simulink model "Electrical_System_2018b_obfs"  (R2019b)
settings: Solver=VariableStepAuto  StartTime=0.0  StopTime=5  RelTol=1e-3  AbsTol=1e-3  EnableMultiTasking=on
InitFcn:
  | Steady_State_Initialisation;
StopFcn:
  | %sscexplore(simlog);
  | %Logging
undefined symbols (not defined in the file): abrlhklxvp, aexgmhuedq, afmfmjnutg, afpphrjpnc, ahuxbyvruc, alarvljztt, amxnyqmnuw, aodrlwvqie, aolhmuplyq, aqpmguuqkg, auesgwirzl, aurophlnng, awamelrhru, ayfhvxflxn, azxkacuhqc, babszerikg, bawhdqanwq, bevoqecvei, bltjvqbchx, bmqsuewujl, bsmyqjfgnf, btvjbsmnve, bywgxqeadw, bziaduxaer, bzmcmdqocb, bzsvyvetat, ccsjnrbsih, cdvenygxwh, cedkrnslhx, cjheorclzs, cjrdshrtqx, ckhavyhcza, ckxewznhlz, cmrcgyiplk, conenicnws, cqkejbgjnn, csfnuwymhe, cunupkhwbh, cwzfvzuxxh, dcadmadufn, dcfponivnv, ddtrqjrhjn, dfhoxvkqas, dfrhtcwpne, dfvomcagjv, djijwylxea, dnmeqksrrm, dnzewbdkaa, dsqcykyxav, dtswwlttmm, ecumpidjtv, edegaywrct, ejjjsmnejc, eknqnehjdz, emvdetzouf, esxbqkbahr, etnkkbreiq, eunoiiiirw, ewewcuedir, fatkfxdhtc ... (+386)
libraries: fl_lib x802, ee_lib x362, fl_ps_legacy_lib x160, nesl_utility x85
(part 2 of 26)

== system Electrical_System_2018b_obfs/Redacted_1221/Redacted_346/Redacted_6610 ==
  Redacted_3546 : Inport
  Redacted_2515 : SimscapeBus  HierarchyStrings=Redacted_600;Redacted_800;Redacted_9392;Redacted_4467
  Redacted_2835 : Subsystem  VariantControlMode=Label  Variant=on  VariantControl=Variant1  LabelModeActiveChoice=Choice
  Redacted_4977 : SimscapeBus  HierarchyStrings=Redacted_3183
  Redacted_8751 : SimscapeBus  HierarchyStrings=Redacted_4818
  Redacted_9208 : SimscapeBus  HierarchyStrings=Redacted_5646;Redacted_1726
  Redacted_995 : SimscapeBus  HierarchyStrings=Redacted_3018;Redacted_5170;Redacted_146
  Redacted_2253 : PMIOPort  Side=Left
  Redacted_1746 : Outport
  wires:
  Redacted_3546/1 -> Redacted_2835/1(Redacted_1740)
  Redacted_2835/1(Redacted_5993) -> Redacted_1746/1
  connections:
  Redacted_2515/LConn3 -- Redacted_9208/RConn1
  Redacted_2515/LConn1 -- Redacted_4977/RConn1
  Redacted_995/RConn1 -- Redacted_2515/LConn4
  Redacted_2253/RConn1 -- Redacted_2515/RConn1
  Redacted_9208/LConn2 -- Redacted_2835/LConn4
  Redacted_8751/LConn1 -- Redacted_2835/LConn2
  Redacted_2515/LConn2 -- Redacted_8751/RConn1
  Redacted_995/LConn1 -- Redacted_2835/RConn1
  Redacted_9208/LConn1 -- Redacted_2835/LConn3
  Redacted_4977/LConn1 -- Redacted_2835/LConn1
  Redacted_995/LConn3 -- Redacted_2835/RConn3
  Redacted_995/LConn2 -- Redacted_2835/RConn2

== system Electrical_System_2018b_obfs/Redacted_1221/Redacted_7523/Redacted_2432 ==
  Redacted_3217 : Inport
  Redacted_3397 : Subsystem  VariantControlMode=Label  Variant=on  VariantControl=Variant1  LabelModeActiveChoice=Choice
  Redacted_4698 : SimscapeBus  HierarchyStrings=Redacted_3957;Redacted_2283
  Redacted_558 : SimscapeBus  HierarchyStrings=Redacted_3;Redacted_3627
  Redacted_672 : SimscapeBus  HierarchyStrings=Redacted_5659;Redacted_4345;Redacted_6835
  Redacted_3110 : PMIOPort  Side=Left
  Redacted_9205 : Outport
  wires:
  Redacted_3217/1 -> Redacted_3397/1(Redacted_7824)
  Redacted_3397/1(Redacted_3107) -> Redacted_9205/1
  connections:
  Redacted_672/LConn1 -- Redacted_3397/RConn1
  Redacted_3397/LConn2 -- Redacted_558/LConn2
  Redacted_672/LConn3 -- Redacted_3397/RConn3
  Redacted_3397/LConn1 -- Redacted_558/LConn1
  Redacted_672/LConn2 -- Redacted_3397/RConn2
  Redacted_4698/LConn1 -- Redacted_558/RConn1
  Redacted_4698/LConn2 -- Redacted_672/RConn1
  Redacted_4698/RConn1 -- Redacted_3110/RConn1

== system Electrical_System_2018b_obfs/Redacted_1221/Redacted_7523/Redacted_5456 ==
  Redacted_8021 : Inport
  Redacted_1170 : Subsystem  VariantControlMode=Label  Variant=on  VariantControl=Variant1  LabelModeActiveChoice=Choice
  Redacted_1204 : SimscapeBus  HierarchyStrings=Redacted_6397
  Redacted_2158 : SimscapeBus  HierarchyStrings=Redacted_1826;Redacted_8420;Redacted_7159
  Redacted_6920 : SimscapeBus  HierarchyStrings=Redacted_4449;Redacted_3882
  Redacted_8170 : SimscapeBus  HierarchyStrings=Redacted_9228
  Redacted_9627 : SimscapeBus  HierarchyStrings=Redacted_8942;Redacted_3488;Redacted_7360;Redacted_9767
  Redacted_2988 : PMIOPort  Side=Left
  Redacted_3690 : Outport
  wires:
  Redacted_8021/1 -> Redacted_1170/1(Redacted_533)
  Redacted_1170/1(Redacted_7763) -> Redacted_3690/1
  connections:
  Redacted_9627/RConn1 -- Redacted_2988/RConn1
  Redacted_1170/LConn3 -- Redacted_6920/LConn1
  Redacted_1170/RConn2 -- Redacted_2158/LConn2
  Redacted_1170/LConn1 -- Redacted_8170/LConn1
  Redacted_1170/RConn3 -- Redacted_2158/LConn3
  Redacted_1170/LConn2 -- Redacted_1204/LConn1
  Redacted_1170/RConn1 -- Redacted_2158/LConn1
  Redacted_1170/LConn4 -- Redacted_6920/LConn2
  Redacted_9627/LConn1 -- Redacted_8170/RConn1
  Redacted_9627/LConn2 -- Redacted_1204/RConn1
  Redacted_9627/LConn3 -- Redacted_6920/RConn1
  Redacted_2158/RConn1 -- Redacted_9627/LConn4

== system Electrical_System_2018b_obfs/Redacted_1221/Redacted_7523/Redacted_5495 ==
  Redacted_4129 : Inport
  Redacted_1590 : SimscapeBus  HierarchyStrings=Redacted_4201;Redacted_9003;Redacted_1739;Redacted_5428
  Redacted_2272 : SimscapeBus  HierarchyStrings=Redacted_9234
  Redacted_2383 : SimscapeBus  HierarchyStrings=Redacted_6746;Redacted_4242;Redacted_8
  Redacted_794 : Subsystem  VariantControlMode=Label  Variant=on  VariantControl=Variant1  LabelModeActiveChoice=Choice
  Redacted_8177 : SimscapeBus  HierarchyStrings=Redacted_1099
  Redacted_9332 : SimscapeBus  HierarchyStrings=Redacted_5631;Redacted_7132
  Redacted_391 : PMIOPort  Side=Left
  Redacted_3176 : Outport
  wires:
  Redacted_4129/1 -> Redacted_794/1(Redacted_2518)
  Redacted_794/1(Redacted_6500) -> Redacted_3176/1
  connections:
  Redacted_1590/LConn3 -- Redacted_9332/RConn1
  Redacted_1590/LConn1 -- Redacted_2272/RConn1
  Redacted_2383/RConn1 -- Redacted_1590/LConn4
  Redacted_391/RConn1 -- Redacted_1590/RConn1
  Redacted_9332/LConn2 -- Redacted_794/LConn4
  Redacted_8177/LConn1 -- Redacted_794/LConn2
  Redacted_1590/LConn2 -- Redacted_8177/RConn1
  Redacted_2383/LConn1 -- Redacted_794/RConn1
  Redacted_9332/LConn1 -- Redacted_794/LConn3
  Redacted_2272/LConn1 -- Redacted_794/LConn1
  Redacted_2383/LConn3 -- Redacted_794/RConn3
  Redacted_2383/LConn2 -- Redacted_794/RConn2

== system Electrical_System_2018b_obfs/Redacted_1221/Redacted_7523/Redacted_6578 ==
  Redacted_753 : Inport
  Redacted_3467 : SimscapeBus  HierarchyStrings=Redacted_171;Redacted_7854
  Redacted_4285 : Subsystem  VariantControlMode=Label  Variant=on  VariantControl=Variant1  LabelModeActiveChoice=Variant1
  Redacted_6843 : SimscapeBus  HierarchyStrings=Redacted_6362;Redacted_5590;Redacted_3762;Redacted_3483;Redacted_686;Redacted_7306;Redacted_1915;Redacted_3972
  Redacted_8097 : SimscapeBus  HierarchyStrings=Redacted_6918;Redacted_8095
  Redacted_3223 : PMIOPort  Side=Left
  Redacted_9705 : Outport
  wires:
  Redacted_753/1 -> Redacted_4285/1(Redacted_4594)
  Redacted_4285/1(Redacted_2646) -> Redacted_9705/1
  connections:
  Redacted_4285/LConn5 -- Redacted_6843/LConn6
  Redacted_3467/LConn1 -- Redacted_4285/LConn1
  Redacted_4285/LConn3 -- Redacted_6843/LConn8
  Redacted_6843/LConn2 -- Redacted_4285/RConn2
  Redacted_4285/LConn6 -- Redacted_6843/LConn5
  Redacted_3467/LConn2 -- Redacted_4285/LConn2
  Redacted_4285/LConn4 -- Redacted_6843/LConn7
  Redacted_6843/LConn1 -- Redacted_4285/RConn1
  Redacted_6843/LConn3 -- Redacted_4285/RConn3
  Redacted_4285/RConn4 -- Redacted_6843/LConn4
  Redacted_8097/LConn2 -- Redacted_6843/RConn1
  Redacted_8097/LConn1 -- Redacted_3467/RConn1
  Redacted_8097/RConn1 -- Redacted_3223/RConn1

== system Electrical_System_2018b_obfs/Redacted_1221/Redacted_7996/Redacted_1 ==
  Redacted_5759 : Inport
  Redacted_2550 : SimscapeBus  HierarchyStrings=Redacted_9618;Redacted_4736
  Redacted_3408 : SimscapeBus  HierarchyStrings=Redacted_1645;Redacted_1267;Redacted_9239;Redacted_9750;Redacted_2245;Redacted_273;Redacted_7118;Redacted_512;Redacted_9809;Redacted_8655;Redacted_936;Redacted_8903;Redacted_7027;Redacted_2453;Redacted_972;Redacted_5288;Redacted_8936;Redacted_9531;Redacted_1783;Redacted_8874;Redacted_9030;Redacted_9120;Redacted_4250;Redacted_7101;Redacted_1578;Redacted_9542;Redacted_8423;Redacted_564;Redacted_4281;Redacted_5468;Redacted_3178;Redacted_328;Redacted_8353;Redacted_293;Redacted_8011;Redacted_7574;Redacted_3943;Redacted_8035;Redacted_1472;Redacted_2571;Redacted_9409;Redacted_7767;Redacted_2428;Redacted_1775;Redacted_6878;Redacted_6039;Redacted_5631;Redacted_9047;Redacted_6076
  Redacted_4377 : Subsystem  VariantControlMode=Label  Variant=on  VariantControl=Variant1  LabelModeActiveChoice=Variant4
  Redacted_8912 : BusSelector  OutputSignals=signal1,signal2,signal3,signal4,signal5,signal6,signal7,signal8,signal9,signal10,signal11,signal12,signal13,signal14,signal15,signal16,signal17,signal18,signal19,signal20,signal21,signal22,signal23,signal24
  Redacted_9300 : SimscapeBus  HierarchyStrings=Redacted_6695;Redacted_8811;Redacted_4024;Redacted_6812;Redacted_1080;Redacted_4478;Redacted_4882;Redacted_900;Redacted_1829;Redacted_7949;Redacted_6769;Redacted_9961;Redacted_3619;Redacted_8591;Redacted_4002;Redacted_4612;Redacted_7888;Redacted_7199;Redacted_4226;Redacted_1876;Redacted_4026;Redacted_5676;Redacted_550;Redacted_3264
  Redacted_9946 : PMIOPort  Side=Left
  Redacted_8821 : PMIOPort  Port=2  Side=Right
  Redacted_8480 : PMIOPort  Port=3  Side=Right
  Redacted_2579 : PMIOPort  Port=4  Side=Right
  Redacted_4777 : Outport
  wires:
  Redacted_8912/13 -> Redacted_4377/13(Redacted_310)  "<signal13>"
  Redacted_8912/14 -> Redacted_4377/14(Redacted_3079)  "<signal14>"
  Redacted_8912/5 -> Redacted_4377/5(Redacted_6798)  "<signal5>"
  Redacted_8912/12 -> Redacted_4377/12(Redacted_6586)  "<signal12>"
  Redacted_8912/6 -> Redacted_4377/6(Redacted_2583)  "<signal6>"
  Redacted_8912/10 -> Redacted_4377/10(Redacted_8855)  "<signal10>"
  Redacted_8912/9 -> Redacted_4377/9(Redacted_970)  "<signal9>"
  Redacted_8912/2 -> Redacted_4377/2(Redacted_5838)  "<signal2>"
  Redacted_8912/16 -> Redacted_4377/16(Redacted_2310)  "<signal16>"
  Redacted_8912/11 -> Redacted_4377/11(Redacted_968)  "<signal11>"
  Redacted_8912/4 -> Redacted_4377/4(Redacted_5102)  "<signal4>"
  Redacted_8912/7 -> Redacted_4377/7(Redacted_1780)  "<signal7>"
  Redacted_5759/1 -> Redacted_8912/1
  Redacted_8912/8 -> Redacted_4377/8(Redacted_5045)  "<signal8>"
  Redacted_8912/3 -> Redacted_4377/3(Redacted_3185)  "<signal3>"
  Redacted_8912/1 -> Redacted_4377/1(Redacted_6515)  "<signal1>"
  Redacted_8912/15 -> Redacted_4377/15(Redacted_2830)  "<signal15>"
  Redacted_8912/17 -> Redacted_4377/17(Redacted_4631)  "<signal17>"
  Redacted_8912/18 -> Redacted_4377/18(Redacted_9555)  "<signal18>"
  Redacted_8912/19 -> Redacted_4377/19(Redacted_7717)  "<signal19>"
  Redacted_8912/20 -> Redacted_4377/20(Redacted_8172)  "<signal20>"
  Redacted_8912/21 -> Redacted_4377/21(Redacted_9013)  "<signal21>"
  Redacted_8912/22 -> Redacted_4377/22(Redacted_7477)  "<signal22>"
  Redacted_8912/23 -> Redacted_4377/23(Redacted_1693)  "<signal23>"
  Redacted_8912/24 -> Redacted_4377/24(Redacted_9125)  "<signal24>"
  connections:
  Redacted_4377/RConn12 -- Redacted_3408/LConn12
  Redacted_4377/RConn7 -- Redacted_3408/LConn7
  Redacted_4377/RConn19 -- Redacted_3408/LConn19
  Redacted_4377/RConn11 -- Redacted_3408/LConn11
  Redacted_4377/RConn28 -- Redacted_3408/LConn28
  Redacted_4377/RConn26 -- Redacted_3408/LConn26
  Redacted_8821/RConn1 -- Redacted_4377/RConn50
  Redacted_4377/RConn27 -- Redacted_3408/LConn27
  Redacted_4377/RConn22 -- Redacted_3408/LConn22
  Redacted_3408/LConn31 -- Redacted_4377/RConn31
  Redacted_4377/RConn29 -- Redacted_3408/LConn29
  Redacted_4377/RConn8 -- Redacted_3408/LConn8
  Redacted_4377/RConn9 -- Redacted_3408/LConn9
  Redacted_4377/RConn6 -- Redacted_3408/LConn6
  Redacted_4377/RConn13 -- Redacted_3408/LConn13
  Redacted_4377/RConn14 -- Redacted_3408/LConn14
  Redacted_4377/RConn24 -- Redacted_3408/LConn24
  Redacted_4377/RConn15 -- Redacted_3408/LConn15
  Redacted_4377/RConn20 -- Redacted_3408/LConn20
  Redacted_4377/RConn10 -- Redacted_3408/LConn10
  Redacted_4377/RConn17 -- Redacted_3408/LConn17
  Redacted_4377/RConn18 -- Redacted_3408/LConn18
  Redacted_4377/RConn16 -- Redacted_3408/LConn16
  Redacted_4377/RConn5 -- Redacted_3408/LConn5
  Redacted_4377/RConn21 -- Redacted_3408/LConn21
  Redacted_3408/LConn30 -- Redacted_4377/RConn30
  Redacted_4377/RConn25 -- Redacted_3408/LConn25
  Redacted_4377/RConn23 -- Redacted_3408/LConn23
  Redacted_4377/RConn52 -- Redacted_2579/RConn1
  Redacted_4377/RConn51 -- Redacted_8480/RConn1
  Redacted_3408/LConn4 -- Redacted_4377/RConn4
  Redacted_3408/LConn2 -- Redacted_4377/RConn2
  Redacted_3408/LConn3 -- Redacted_4377/RConn3
  Redacted_3408/LConn1 -- Redacted_4377/RConn1
  Redacted_3408/RConn1 -- Redacted_2550/LConn2
  Redacted_9946/RConn1 -- Redacted_2550/RConn1
  Redacted_9300/LConn1 -- Redacted_4377/LConn1
  Redacted_9300/LConn2 -- Redacted_4377/LConn2
  Redacted_9300/LConn3 -- Redacted_4377/LConn3
  Redacted_9300/LConn4 -- Redacted_4377/LConn4
  Redacted_9300/LConn5 -- Redacted_4377/LConn5
  Redacted_9300/LConn6 -- Redacted_4377/LConn6
  Redacted_9300/LConn7 -- Redacted_4377/LConn7
  Redacted_9300/LConn8 -- Redacted_4377/LConn8
  Redacted_9300/LConn9 -- Redacted_4377/LConn9
  Redacted_9300/LConn10 -- Redacted_4377/LConn10
  Redacted_9300/LConn11 -- Redacted_4377/LConn11
  Redacted_9300/LConn12 -- Redacted_4377/LConn12
  Redacted_9300/LConn13 -- Redacted_4377/LConn13
  Redacted_9300/LConn14 -- Redacted_4377/LConn14
  Redacted_9300/LConn15 -- Redacted_4377/LConn15
  Redacted_9300/LConn16 -- Redacted_4377/LConn16
  Redacted_2550/LConn1 -- Redacted_9300/RConn1
  Redacted_9300/LConn18 -- Redacted_4377/LConn18
  Redacted_9300/LConn19 -- Redacted_4377/LConn19
  Redacted_9300/LConn17 -- Redacted_4377/LConn17
  Redacted_9300/LConn20 -- Redacted_4377/LConn20
  Redacted_9300/LConn21 -- Redacted_4377/LConn21
  Redacted_9300/LConn22 -- Redacted_4377/LConn22
  Redacted_9300/LConn23 -- Redacted_4377/LConn23
  Redacted_9300/LConn24 -- Redacted_4377/LConn24
  Redacted_3408/LConn32 -- Redacted_4377/RConn32
  Redacted_3408/LConn33 -- Redacted_4377/RConn33
  Redacted_3408/LConn34 -- Redacted_4377/RConn34
  Redacted_3408/LConn35 -- Redacted_4377/RConn35
  Redacted_3408/LConn36 -- Redacted_4377/RConn36
  Redacted_3408/LConn37 -- Redacted_4377/RConn37
  Redacted_3408/LConn38 -- Redacted_4377/RConn38
  Redacted_3408/LConn39 -- Redacted_4377/RConn39
  Redacted_3408/LConn40 -- Redacted_4377/RConn40
  Redacted_3408/LConn41 -- Redacted_4377/RConn41
  Redacted_3408/LConn42 -- Redacted_4377/RConn42
  Redacted_3408/LConn43 -- Redacted_4377/RConn43
  Redacted_3408/LConn44 -- Redacted_4377/RConn44
  Redacted_3408/LConn45 -- Redacted_4377/RConn45
  Redacted_3408/LConn46 -- Redacted_4377/RConn46
  Redacted_3408/LConn47 -- Redacted_4377/RConn47
  Redacted_3408/LConn48 -- Redacted_4377/RConn48
  Redacted_4377/RConn49 -- Redacted_3408/LConn49

== system Electrical_System_2018b_obfs/Redacted_1221/Redacted_7996/Redacted_2 ==
  Redacted_9139 : Inport
  Redacted_2321 : SimscapeBus  HierarchyStrings=Redacted_9740;Redacted_2584
  Redacted_3302 : SimscapeBus  HierarchyStrings=Redacted_3734;Redacted_3790;Redacted_712;Redacted_9760;Redacted_78;Redacted_8266
  Redacted_38 : Subsystem  VariantControlMode=Label  Variant=on  VariantControl=Variant1  LabelModeActiveChoice=Variant1
  Redacted_6014 : SimscapeBus  HierarchyStrings=Redacted_7779;Redacted_9774;Redacted_1058;Redacted_9808;Redacted_661;Redacted_3856;Redacted_607;Redacted_1221;Redacted_8690;Redacted_6084
  Redacted_6226 : BusSelector  OutputSignals=signal25,signal26,signal27,signal28,signal29,signal30
  Redacted_7352 : PMIOPort  Side=Left
  Redacted_3930 : PMIOPort  Port=2  Side=Right
  Redacted_7448 : PMIOPort  Port=3  Side=Right
  Redacted_3058 : PMIOPort  Port=4  Side=Right
  Redacted_9760 : PMIOPort  Port=5  Side=Right
  Redacted_7172 : PMIOPort  Port=6  Side=Right
  Redacted_5489 : PMIOPort  Port=7  Side=Right
  Redacted_9750 : Outport
  wires:
  Redacted_6226/5 -> Redacted_38/5(Redacted_9135)  "<signal29>"
  Redacted_6226/2 -> Redacted_38/2(Redacted_9730)  "<signal26>"
  Redacted_9139/1 -> Redacted_6226/1
  Redacted_6226/1 -> Redacted_38/1(Redacted_7517)  "<signal25>"
  Redacted_6226/6 -> Redacted_38/6(Redacted_9726)  "<signal30>"
  Redacted_6226/3 -> Redacted_38/3(Redacted_3026)  "<signal27>"
  Redacted_6226/4 -> Redacted_38/4(Redacted_8427)  "<signal28>"
  connections:
  Redacted_7352/RConn1 -- Redacted_2321/RConn1
  Redacted_2321/LConn2 -- Redacted_3302/RConn1
  Redacted_2321/LConn1 -- Redacted_6014/RConn1
  Redacted_3302/LConn6 -- Redacted_38/LConn16
  Redacted_3302/LConn5 -- Redacted_38/LConn15
  Redacted_3302/LConn4 -- Redacted_38/LConn14
  Redacted_3302/LConn3 -- Redacted_38/LConn13
  Redacted_3302/LConn2 -- Redacted_38/LConn12
  Redacted_3302/LConn1 -- Redacted_38/LConn11
  Redacted_38/RConn6 -- Redacted_5489/RConn1
  Redacted_7172/RConn1 -- Redacted_38/RConn5
  Redacted_7448/RConn1 -- Redacted_38/RConn2
  Redacted_3930/RConn1 -- Redacted_38/RConn3
  Redacted_38/RConn1 -- Redacted_3058/RConn1
  Redacted_38/RConn4 -- Redacted_9760/RConn1
  Redacted_6014/LConn5 -- Redacted_38/LConn5
  Redacted_6014/LConn3 -- Redacted_38/LConn3
  Redacted_6014/LConn6 -- Redacted_38/LConn6
  Redacted_6014/LConn4 -- Redacted_38/LConn4
  Redacted_6014/LConn1 -- Redacted_38/LConn1
  Redacted_6014/LConn2 -- Redacted_38/LConn2
  Redacted_38/LConn7 -- Redacted_6014/LConn7
  Redacted_38/LConn10 -- Redacted_6014/LConn10
  Redacted_38/LConn9 -- Redacted_6014/LConn9
  Redacted_38/LConn8 -- Redacted_6014/LConn8

== system Electrical_System_2018b_obfs/Redacted_1221/Redacted_7996/Redacted_7418 ==
  Redacted_5759 : Inport
  Redacted_2550 : SimscapeBus  HierarchyStrings=Redacted_9618;Redacted_4736
  Redacted_3408 : SimscapeBus  HierarchyStrings=Redacted_1645;Redacted_1267;Redacted_9239;Redacted_9750;Redacted_2245;Redacted_273;Redacted_7118;Redacted_512;Redacted_9809;Redacted_8655;Redacted_936;Redacted_8903;Redacted_7027;Redacted_2453;Redacted_972;Redacted_5288;Redacted_8936;Redacted_9531;Redacted_1783;Redacted_8874;Redacted_9030;Redacted_9120;Redacted_4250;Redacted_7101;Redacted_1578;Redacted_9542;Redacted_8423;Redacted_564;Redacted_4281;Redacted_5468;Redacted_3178;Redacted_328;Redacted_8353;Redacted_293;Redacted_8011;Redacted_7574;Redacted_3943;Redacted_8035;Redacted_1472;Redacted_2571;Redacted_9409;Redacted_7767;Redacted_2428;Redacted_1775;Redacted_6878;Redacted_6039;Redacted_5631;Redacted_9047;Redacted_6076
  Redacted_4377 : Subsystem  VariantControlMode=Label  Variant=on  VariantControl=Variant1  LabelModeActiveChoice=Variant4
  Redacted_8912 : BusSelector  OutputSignals=signal1,signal2,signal3,signal4,signal5,signal6,signal7,signal8,signal9,signal10,signal11,signal12,signal13,signal14,signal15,signal16,signal17,signal18,signal19,signal20,signal21,signal22,signal23,signal24
  Redacted_9300 : SimscapeBus  HierarchyStrings=Redacted_6695;Redacted_8811;Redacted_4024;Redacted_6812;Redacted_1080;Redacted_4478;Redacted_4882;Redacted_900;Redacted_1829;Redacted_7949;Redacted_6769;Redacted_9961;Redacted_3619;Redacted_8591;Redacted_4002;Redacted_4612;Redacted_7888;Redacted_7199;Redacted_4226;Redacted_1876;Redacted_4026;Redacted_5676;Redacted_550;Redacted_3264
  Redacted_9946 : PMIOPort  Side=Left
  Redacted_8821 : PMIOPort  Port=2  Side=Right
  Redacted_8480 : PMIOPort  Port=3  Side=Right
  Redacted_2579 : PMIOPort  Port=4  Side=Right
  Redacted_4777 : Outport
  wires:
  Redacted_8912/13 -> Redacted_4377/13(Redacted_310)  "<signal13>"
  Redacted_8912/14 -> Redacted_4377/14(Redacted_3079)  "<signal14>"
  Redacted_8912/5 -> Redacted_4377/5(Redacted_6798)  "<signal5>"
  Redacted_8912/12 -> Redacted_4377/12(Redacted_6586)  "<signal12>"
  Redacted_8912/6 -> Redacted_4377/6(Redacted_2583)  "<signal6>"
  Redacted_8912/10 -> Redacted_4377/10(Redacted_8855)  "<signal10>"
  Redacted_8912/9 -> Redacted_4377/9(Redacted_970)  "<signal9>"
  Redacted_8912/2 -> Redacted_4377/2(Redacted_5838)  "<signal2>"
  Redacted_8912/16 -> Redacted_4377/16(Redacted_2310)  "<signal16>"
  Redacted_8912/11 -> Redacted_4377/11(Redacted_968)  "<signal11>"
  Redacted_8912/4 -> Redacted_4377/4(Redacted_5102)  "<signal4>"
  Redacted_8912/7 -> Redacted_4377/7(Redacted_1780)  "<signal7>"
  Redacted_5759/1 -> Redacted_8912/1
  Redacted_8912/8 -> Redacted_4377/8(Redacted_5045)  "<signal8>"
  Redacted_8912/3 -> Redacted_4377/3(Redacted_3185)  "<signal3>"
  Redacted_8912/1 -> Redacted_4377/1(Redacted_6515)  "<signal1>"
  Redacted_8912/15 -> Redacted_4377/15(Redacted_2830)  "<signal15>"
  Redacted_8912/17 -> Redacted_4377/17(Redacted_4631)  "<signal17>"
  Redacted_8912/18 -> Redacted_4377/18(Redacted_9555)  "<signal18>"
  Redacted_8912/19 -> Redacted_4377/19(Redacted_7717)  "<signal19>"
  Redacted_8912/20 -> Redacted_4377/20(Redacted_8172)  "<signal20>"
  Redacted_8912/21 -> Redacted_4377/21(Redacted_9013)  "<signal21>"
  Redacted_8912/22 -> Redacted_4377/22(Redacted_7477)  "<signal22>"
  Redacted_8912/23 -> Redacted_4377/23(Redacted_1693)  "<signal23>"
  Redacted_8912/24 -> Redacted_4377/24(Redacted_9125)  "<signal24>"
  connections:
  Redacted_4377/RConn12 -- Redacted_3408/LConn12
  Redacted_4377/RConn7 -- Redacted_3408/LConn7
  Redacted_4377/RConn19 -- Redacted_3408/LConn19
  Redacted_4377/RConn11 -- Redacted_3408/LConn11
  Redacted_4377/RConn28 -- Redacted_3408/LConn28
  Redacted_4377/RConn26 -- Redacted_3408/LConn26
  Redacted_8821/RConn1 -- Redacted_4377/RConn50
  Redacted_4377/RConn27 -- Redacted_3408/LConn27
  Redacted_4377/RConn22 -- Redacted_3408/LConn22
  Redacted_3408/LConn31 -- Redacted_4377/RConn31
  Redacted_4377/RConn29 -- Redacted_3408/LConn29
  Redacted_4377/RConn8 -- Redacted_3408/LConn8
  Redacted_4377/RConn9 -- Redacted_3408/LConn9
  Redacted_4377/RConn6 -- Redacted_3408/LConn6
  Redacted_4377/RConn13 -- Redacted_3408/LConn13
  Redacted_4377/RConn14 -- Redacted_3408/LConn14
  Redacted_4377/RConn24 -- Redacted_3408/LConn24
  Redacted_4377/RConn15 -- Redacted_3408/LConn15
  Redacted_4377/RConn20 -- Redacted_3408/LConn20
  Redacted_4377/RConn10 -- Redacted_3408/LConn10
  Redacted_4377/RConn17 -- Redacted_3408/LConn17
  Redacted_4377/RConn18 -- Redacted_3408/LConn18
  Redacted_4377/RConn16 -- Redacted_3408/LConn16
  Redacted_4377/RConn5 -- Redacted_3408/LConn5
  Redacted_4377/RConn21 -- Redacted_3408/LConn21
  Redacted_3408/LConn30 -- Redacted_4377/RConn30
  Redacted_4377/RConn25 -- Redacted_3408/LConn25
  Redacted_4377/RConn23 -- Redacted_3408/LConn23
  Redacted_4377/RConn52 -- Redacted_2579/RConn1
  Redacted_4377/RConn51 -- Redacted_8480/RConn1
  Redacted_3408/LConn4 -- Redacted_4377/RConn4
  Redacted_3408/LConn2 -- Redacted_4377/RConn2
  Redacted_3408/LConn3 -- Redacted_4377/RConn3
  Redacted_3408/LConn1 -- Redacted_4377/RConn1
  Redacted_3408/RConn1 -- Redacted_2550/LConn2
  Redacted_9946/RConn1 -- Redacted_2550/RConn1
  Redacted_9300/LConn1 -- Redacted_4377/LConn1
  Redacted_9300/LConn2 -- Redacted_4377/LConn2
  Redacted_9300/LConn3 -- Redacted_4377/LConn3
  Redacted_9300/LConn4 -- Redacted_4377/LConn4
  Redacted_9300/LConn5 -- Redacted_4377/LConn5
  Redacted_9300/LConn6 -- Redacted_4377/LConn6
  Redacted_9300/LConn7 -- Redacted_4377/LConn7
  Redacted_9300/LConn8 -- Redacted_4377/LConn8
  Redacted_9300/LConn9 -- Redacted_4377/LConn9
  Redacted_9300/LConn10 -- Redacted_4377/LConn10
  Redacted_9300/LConn11 -- Redacted_4377/LConn11
  Redacted_9300/LConn12 -- Redacted_4377/LConn12
  Redacted_9300/LConn13 -- Redacted_4377/LConn13
  Redacted_9300/LConn14 -- Redacted_4377/LConn14
  Redacted_9300/LConn15 -- Redacted_4377/LConn15
  Redacted_9300/LConn16 -- Redacted_4377/LConn16
  Redacted_2550/LConn1 -- Redacted_9300/RConn1
  Redacted_9300/LConn18 -- Redacted_4377/LConn18
  Redacted_9300/LConn19 -- Redacted_4377/LConn19
  Redacted_9300/LConn17 -- Redacted_4377/LConn17
  Redacted_9300/LConn20 -- Redacted_4377/LConn20
  Redacted_9300/LConn21 -- Redacted_4377/LConn21
  Redacted_9300/LConn22 -- Redacted_4377/LConn22
  Redacted_9300/LConn23 -- Redacted_4377/LConn23
  Redacted_9300/LConn24 -- Redacted_4377/LConn24
  Redacted_3408/LConn32 -- Redacted_4377/RConn32
  Redacted_3408/LConn33 -- Redacted_4377/RConn33
  Redacted_3408/LConn34 -- Redacted_4377/RConn34
  Redacted_3408/LConn35 -- Redacted_4377/RConn35
  Redacted_3408/LConn36 -- Redacted_4377/RConn36
  Redacted_3408/LConn37 -- Redacted_4377/RConn37
  Redacted_3408/LConn38 -- Redacted_4377/RConn38
  Redacted_3408/LConn39 -- Redacted_4377/RConn39
  Redacted_3408/LConn40 -- Redacted_4377/RConn40
  Redacted_3408/LConn41 -- Redacted_4377/RConn41
  Redacted_3408/LConn42 -- Redacted_4377/RConn42
  Redacted_3408/LConn43 -- Redacted_4377/RConn43
  Redacted_3408/LConn44 -- Redacted_4377/RConn44
  Redacted_3408/LConn45 -- Redacted_4377/RConn45
  Redacted_3408/LConn46 -- Redacted_4377/RConn46
  Redacted_3408/LConn47 -- Redacted_4377/RConn47
  Redacted_3408/LConn48 -- Redacted_4377/RConn48
  Redacted_4377/RConn49 -- Redacted_3408/LConn49

== system Electrical_System_2018b_obfs/Redacted_1221/Redacted_7996/Redacted_9242 ==
  Redacted_9139 : Inport
  Redacted_2321 : SimscapeBus  HierarchyStrings=Redacted_9740;Redacted_2584
  Redacted_3302 : SimscapeBus  HierarchyStrings=Redacted_3734;Redacted_3790;Redacted_712;Redacted_9760;Redacted_78;Redacted_8266
  Redacted_38 : Subsystem  VariantControlMode=Label  Variant=on  VariantControl=Variant1  LabelModeActiveChoice=Variant1
  Redacted_6014 : SimscapeBus  HierarchyStrings=Redacted_7779;Redacted_9774;Redacted_1058;Redacted_9808;Redacted_661;Redacted_3856;Redacted_607;Redacted_1221;Redacted_8690;Redacted_6084
  Redacted_6226 : BusSelector  OutputSignals=signal25,signal26,signal27,signal28,signal29,signal30
  Redacted_7352 : PMIOPort  Side=Left
  Redacted_3930 : PMIOPort  Port=2  Side=Right
  Redacted_7448 : PMIOPort  Port=3  Side=Right
  Redacted_3058 : PMIOPort  Port=4  Side=Right
  Redacted_9760 : PMIOPort  Port=5  Side=Right
  Redacted_7172 : PMIOPort  Port=6  Side=Right
  Redacted_5489 : PMIOPort  Port=7  Side=Right
  Redacted_9750 : Outport
  wires:
  Redacted_6226/4 -> Redacted_38/4(Redacted_8427)  "<signal28>"
  Redacted_6226/3 -> Redacted_38/3(Redacted_3026)  "<signal27>"
  Redacted_6226/6 -> Redacted_38/6(Redacted_9726)  "<signal30>"
  Redacted_6226/1 -> Redacted_38/1(Redacted_7517)  "<signal25>"
  Redacted_9139/1 -> Redacted_6226/1
  Redacted_6226/2 -> Redacted_38/2(Redacted_9730)  "<signal26>"
  Redacted_6226/5 -> Redacted_38/5(Redacted_9135)  "<signal29>"
  connections:
  Redacted_38/LConn8 -- Redacted_6014/LConn8
  Redacted_38/LConn9 -- Redacted_6014/LConn9
  Redacted_38/LConn10 -- Redacted_6014/LConn10
  Redacted_38/LConn7 -- Redacted_6014/LConn7
  Redacted_6014/LConn2 -- Redacted_38/LConn2
  Redacted_6014/LConn1 -- Redacted_38/LConn1
  Redacted_6014/LConn4 -- Redacted_38/LConn4
  Redacted_6014/LConn6 -- Redacted_38/LConn6
  Redacted_6014/LConn3 -- Redacted_38/LConn3
  Redacted_6014/LConn5 -- Redacted_38/LConn5
  Redacted_38/RConn4 -- Redacted_9760/RConn1
  Redacted_38/RConn1 -- Redacted_3058/RConn1
  Redacted_3930/RConn1 -- Redacted_38/RConn3
  Redacted_7448/RConn1 -- Redacted_38/RConn2
  Redacted_7172/RConn1 -- Redacted_38/RConn5
  Redacted_38/RConn6 -- Redacted_5489/RConn1
  Redacted_3302/LConn1 -- Redacted_38/LConn11
  Redacted_3302/LConn2 -- Redacted_38/LConn12
  Redacted_3302/LConn3 -- Redacted_38/LConn13
  Redacted_3302/LConn4 -- Redacted_38/LConn14
  Redacted_3302/LConn5 -- Redacted_38/LConn15
  Redacted_3302/LConn6 -- Redacted_38/LConn16
  Redacted_2321/LConn1 -- Redacted_6014/RConn1
  Redacted_2321/LConn2 -- Redacted_3302/RConn1
  Redacted_7352/RConn1 -- Redacted_2321/RConn1

== system Electrical_System_2018b_obfs/Redacted_1750/Redacted_1925/Redacted_8189 ==
  Redacted_1905 : fl_lib/Electrical/Electrical Sensors/Voltage Sensor
  Redacted_2601 : fl_lib/Physical Signals/Sources/PS Constant  constant=uhqvuawrkj
  Redacted_2736 : fl_ps_legacy_lib/Legacy Physical Signals/Functions/PS Divide
      settings: SourceProductName=Simscape  SourceProductBaseCode=SS  InternalSimscapePortConfiguration="{\"Bottom\":[],\"Left\":[{\"id\":\"I1\",\"label\":\"\",\"type\":\"input\"},{\"id\":\"I2\",\"label\":\"\",\"type\":\"input\"}],\"Right\":[{\"id\":\"O\",\"label\":\"\",\"type\":\"output\"}],\"Top\":[]}"
  Redacted_2889 : fl_lib/Electrical/Electrical Elements/Variable Resistor  Rmin=cdglhkebrb Ohm  i_specify=off  i_priority=None  i=vaqzmbjoip A  i_nominal_specify=off  i_nominal_unit=A  i_nominal_value=oigeomftmz  v_specify=on  v_priority=None  v=zxalaqxdeb V  v_nominal_specify=off  v_nominal_unit=V  v_nominal_value=ghixzyywgw
  Redacted_4175 : fl_ps_legacy_lib/Legacy Physical Signals/Functions/PS Product
      settings: SourceProductName=Simscape  SourceProductBaseCode=SS
  Redacted_4388 : fl_lib/Electrical/Electrical Sensors/Voltage Sensor
  Redacted_565 : fl_lib/Electrical/Electrical Sensors/Voltage Sensor
  Redacted_6220 : fl_lib/Physical Signals/Sources/PS Constant  constant=nzzpdqltsx
  Redacted_6568 : fl_lib/Physical Signals/Sources/PS Constant  constant=wsyaszviyb
  Redacted_6855 : fl_ps_legacy_lib/Legacy Physical Signals/Functions/PS Product
      settings: SourceProductName=Simscape  SourceProductBaseCode=SS
  Redacted_7192 : fl_lib/Electrical/Electrical Elements/Variable Resistor  Rmin=ozjrqvrsoh Ohm  i_specify=off  i_priority=None  i=aotksbjcfm A  i_nominal_specify=off  i_nominal_unit=A  i_nominal_value=pucpayezqy  v_specify=on  v_priority=None  v=vhsdmydpou V  v_nominal_specify=off  v_nominal_unit=V  v_nominal_value=xhuyxhgzwr
  Redacted_8133 : fl_ps_legacy_lib/Legacy Physical Signals/Functions/PS Divide
      settings: SourceProductName=Simscape  SourceProductBaseCode=SS  InternalSimscapePortConfiguration="{\"Bottom\":[],\"Left\":[{\"id\":\"I1\",\"label\":\"\",\"type\":\"input\"},{\"id\":\"I2\",\"label\":\"\",\"type\":\"input\"}],\"Right\":[{\"id\":\"O\",\"label\":\"\",\"type\":\"output\"}],\"Top\":[]}"
  Redacted_8896 : fl_lib/Electrical/Electrical Elements/Variable Resistor  Rmin=idublxdcsh Ohm  i_specify=off  i_priority=None  i=fckqrxyseh A  i_nominal_specify=off  i_nominal_unit=A  i_nominal_value=djtkbnxcfl  v_specify=on  v_priority=None  v=cfxnnzgixn V  v_nominal_specify=off  v_nominal_unit=V  v_nominal_value=wtclrmkntc
  Redacted_8961 : fl_ps_legacy_lib/Legacy Physical Signals/Functions/PS Product
      settings: SourceProductName=Simscape  SourceProductBaseCode=SS
  Redacted_990 : fl_ps_legacy_lib/Legacy Physical Signals/Functions/PS Divide
      settings: SourceProductName=Simscape  SourceProductBaseCode=SS  InternalSimscapePortConfiguration="{\"Bottom\":[],\"Left\":[{\"id\":\"I1\",\"label\":\"\",\"type\":\"input\"},{\"id\":\"I2\",\"label\":\"\",\"type\":\"input\"}],\"Right\":[{\"id\":\"O\",\"label\":\"\",\"type\":\"output\"}],\"Top\":[]}"
  Redacted_191 : PMIOPort  Side=Left
  Redacted_5684 : PMIOPort  Port=2  Side=Left
  Redacted_8638 : PMIOPort  Port=3  Side=Left
  Redacted_2799 : PMIOPort  Port=4  Side=Left
  Redacted_4825 : PMIOPort  Port=5  Side=Left
  Redacted_997 : PMIOPort  Port=6  Side=Left
  connections:
  Redacted_4175/LConn2 -- Redacted_565/RConn1 -- Redacted_4175/LConn1
  Redacted_2889/LConn2 -- Redacted_8638/RConn1 -- Redacted_565/LConn1
  Redacted_565/RConn2 -- Redacted_2799/RConn1 -- Redacted_2889/RConn1
  Redacted_997/RConn1 -- Redacted_1905/RConn2 -- Redacted_8896/RConn1
  Redacted_5684/RConn1 -- Redacted_4388/LConn1 -- Redacted_7192/LConn2
  Redacted_4825/RConn1 -- Redacted_7192/RConn1 -- Redacted_4388/RConn2
  Redacted_191/RConn1 -- Redacted_8896/LConn2 -- Redacted_1905/LConn1
  Redacted_6855/LConn1 -- Redacted_4388/RConn1 -- Redacted_6855/LConn2
  Redacted_8961/LConn2 -- Redacted_1905/RConn1 -- Redacted_8961/LConn1
  Redacted_2736/LConn2 -- Redacted_2601/RConn1
  Redacted_2736/RConn1 -- Redacted_2889/LConn1
  Redacted_4175/RConn1 -- Redacted_2736/LConn1
  Redacted_6855/RConn1 -- Redacted_8133/LConn1
  Redacted_6220/RConn1 -- Redacted_8133/LConn2
  Redacted_8133/RConn1 -- Redacted_7192/LConn1
  Redacted_990/RConn1 -- Redacted_8896/LConn1
  Redacted_8961/RConn1 -- Redacted_990/LConn1
  Redacted_6568/RConn1 -- Redacted_990/LConn2

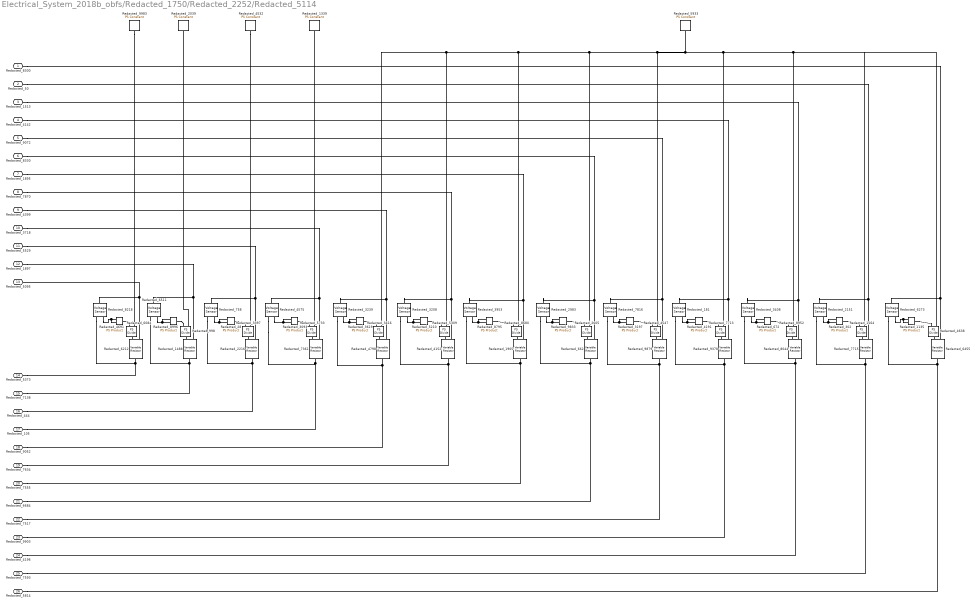
== system Electrical_System_2018b_obfs/Redacted_1750/Redacted_2252/Redacted_5114 ==
  Redacted_{28,302,672,1135,3093,3197,3619,4191,4691,5210,8795,8996,9833} (13 alike) : fl_ps_legacy_lib/Legacy Physical Signals/Functions/PS Product
      settings: SourceProductName=Simscape  SourceProductBaseCode=SS
  Redacted_{998,1164,2605,3397,3416,4547,4638,5309,5733,6084,7713,8680,8952} (13 alike) : fl_ps_legacy_lib/Legacy Physical Signals/Functions/PS Divide
      settings: SourceProductName=Simscape  SourceProductBaseCode=SS  InternalSimscapePortConfiguration="{\"Bottom\":[],\"Left\":[{\"id\":\"I1\",\"label\":\"\",\"type\":\"input\"},{\"id\":\"I2\",\"label\":\"\",\"type\":\"input\"}],\"Right\":[{\"id\":\"O\",\"label\":\"\",\"type\":\"output\"}],\"Top\":[]}"
  Redacted_1339 : fl_lib/Physical Signals/Sources/PS Constant  constant=edmdisnwna
  Redacted_1488 : fl_lib/Electrical/Electrical Elements/Variable Resistor  Rmin=dfcydkdksa Ohm  i_specify=off  i_priority=None  i=zmnqgulykt A  i_nominal_specify=off  i_nominal_unit=A  i_nominal_value=jhatdsscvc  v_specify=off  v_priority=None  v=jvvumrtgyu V  v_nominal_specify=off  v_nominal_unit=V  v_nominal_value=edqbyqqqyv
  Redacted_{181,758,2151,2983,3208,3239,3408,3953,4575,6273,6511,7816,8218} (13 alike) : fl_lib/Electrical/Electrical Sensors/Voltage Sensor
  Redacted_1905 : fl_lib/Electrical/Electrical Elements/Variable Resistor  Rmin=iwypzrktxo Ohm  i_specify=off  i_priority=None  i=ncdbuzteqy A  i_nominal_specify=off  i_nominal_unit=A  i_nominal_value=vobpjmtmno  v_specify=off  v_priority=None  v=qwokqqbmqg V  v_nominal_specify=off  v_nominal_unit=V  v_nominal_value=lalscjvjas
  Redacted_2039 : fl_lib/Physical Signals/Sources/PS Constant  constant=fifxzkdgdp
  Redacted_2216 : fl_lib/Electrical/Electrical Elements/Variable Resistor  Rmin=mxavilupid Ohm  i_specify=off  i_priority=None  i=ckhsgvbaho A  i_nominal_specify=off  i_nominal_unit=A  i_nominal_value=vxiiwizwpa  v_specify=off  v_priority=None  v=ncrrdjxnlp V  v_nominal_specify=off  v_nominal_unit=V  v_nominal_value=pewvnuuxhh
  Redacted_4152 : fl_lib/Electrical/Electrical Elements/Variable Resistor  Rmin=wsblmwhexu Ohm  i_specify=off  i_priority=None  i=wsuibmqosd A  i_nominal_specify=off  i_nominal_unit=A  i_nominal_value=khapnkjori  v_specify=off  v_priority=None  v=dnmekudang V  v_nominal_specify=off  v_nominal_unit=V  v_nominal_value=nmdzgkfmfb
  Redacted_4532 : fl_lib/Physical Signals/Sources/PS Constant  constant=fiayfacgyn
  Redacted_4798 : fl_lib/Electrical/Electrical Elements/Variable Resistor  Rmin=zdfvqdpapy Ohm  i_specify=off  i_priority=None  i=ucpuohmbqp A  i_nominal_specify=off  i_nominal_unit=A  i_nominal_value=nbmhghjcne  v_specify=off  v_priority=None  v=oesrmxltex V  v_nominal_specify=off  v_nominal_unit=V  v_nominal_value=utdeukrase
  Redacted_5933 : fl_lib/Physical Signals/Sources/PS Constant  constant=djpjerokjs
  Redacted_6212 : fl_lib/Electrical/Electrical Elements/Variable Resistor  Rmin=jdftespkns Ohm  i_specify=off  i_priority=None  i=vmimntkzkj A  i_nominal_specify=off  i_nominal_unit=A  i_nominal_value=ptzbppokiy  v_specify=off  v_priority=None  v=glaxpchapx V  v_nominal_specify=off  v_nominal_unit=V  v_nominal_value=fnkikuzjii
  Redacted_6455 : fl_lib/Electrical/Electrical Elements/Variable Resistor  Rmin=fnohzigxlv Ohm  i_specify=off  i_priority=None  i=otschantrv A  i_nominal_specify=off  i_nominal_unit=A  i_nominal_value=fefbermykw  v_specify=off  v_priority=None  v=yrbpgkfypq V  v_nominal_specify=off  v_nominal_unit=V  v_nominal_value=wjncberkeu
  Redacted_662 : fl_lib/Electrical/Electrical Elements/Variable Resistor  Rmin=akjyvdypop Ohm  i_specify=off  i_priority=None  i=jrwxzovdud A  i_nominal_specify=off  i_nominal_unit=A  i_nominal_value=fficgxnlsk  v_specify=off  v_priority=None  v=zxniwbkknj V  v_nominal_specify=off  v_nominal_unit=V  v_nominal_value=lpwbvgybkp
  Redacted_7361 : fl_lib/Electrical/Electrical Elements/Variable Resistor  Rmin=lxsewpxtzv Ohm  i_specify=off  i_priority=None  i=hklinaiatu A  i_nominal_specify=off  i_nominal_unit=A  i_nominal_value=tcjbxqatef  v_specify=off  v_priority=None  v=hrjesjsxhd V  v_nominal_specify=off  v_nominal_unit=V  v_nominal_value=osrmdutjac
  Redacted_7715 : fl_lib/Electrical/Electrical Elements/Variable Resistor  Rmin=swtyihlaps Ohm  i_specify=off  i_priority=None  i=wtpfckeixv A  i_nominal_specify=off  i_nominal_unit=A  i_nominal_value=jstpxzyzzb  v_specify=off  v_priority=None  v=xxxjteruxl V  v_nominal_specify=off  v_nominal_unit=V  v_nominal_value=vlpvwrnitf
  Redacted_8044 : fl_lib/Electrical/Electrical Elements/Variable Resistor  Rmin=ugoygponad Ohm  i_specify=off  i_priority=None  i=eoefpaxguw A  i_nominal_specify=off  i_nominal_unit=A  i_nominal_value=kbuxstggxe  v_specify=off  v_priority=None  v=ngyijhtmwb V  v_nominal_specify=off  v_nominal_unit=V  v_nominal_value=ytmjjijjtg
  Redacted_9378 : fl_lib/Electrical/Electrical Elements/Variable Resistor  Rmin=mzcufwlirv Ohm  i_specify=off  i_priority=None  i=twurhntrwt A  i_nominal_specify=off  i_nominal_unit=A  i_nominal_value=ywcjlbkjjz  v_specify=off  v_priority=None  v=jjknhxffqr V  v_nominal_specify=off  v_nominal_unit=V  v_nominal_value=femmaspdtf
  Redacted_9879 : fl_lib/Electrical/Electrical Elements/Variable Resistor  Rmin=fjkslvbgmn Ohm  i_specify=off  i_priority=None  i=jmzwpbirsb A  i_nominal_specify=off  i_nominal_unit=A  i_nominal_value=ryykwkawdp  v_specify=off  v_priority=None  v=zkiomjxauo V  v_nominal_specify=off  v_nominal_unit=V  v_nominal_value=tefzuyowwk
  Redacted_9983 : fl_lib/Physical Signals/Sources/PS Constant  constant=ceaojbxbhc
  Redacted_8300 : PMIOPort  Side=Left
  Redacted_50 : PMIOPort  Port=2  Side=Left
  Redacted_1513 : PMIOPort  Port=3  Side=Left
  Redacted_4142 : PMIOPort  Port=4  Side=Left
  Redacted_9072 : PMIOPort  Port=5  Side=Left
  Redacted_8330 : PMIOPort  Port=6  Side=Left
  Redacted_1895 : PMIOPort  Port=7  Side=Left
  Redacted_7870 : PMIOPort  Port=8  Side=Left
  Redacted_4399 : PMIOPort  Port=9  Side=Left
  Redacted_3718 : PMIOPort  Port=10  Side=Left
  Redacted_5529 : PMIOPort  Port=11  Side=Left
  Redacted_1897 : PMIOPort  Port=12  Side=Left
  Redacted_5095 : PMIOPort  Port=13  Side=Left
  Redacted_5373 : PMIOPort  Port=14  Side=Left
  Redacted_7138 : PMIOPort  Port=15  Side=Left
  Redacted_444 : PMIOPort  Port=16  Side=Left
  Redacted_105 : PMIOPort  Port=17  Side=Left
  Redacted_9052 : PMIOPort  Port=18  Side=Left
  Redacted_7634 : PMIOPort  Port=19  Side=Left
  Redacted_7555 : PMIOPort  Port=20  Side=Left
  Redacted_6684 : PMIOPort  Port=21  Side=Left
  Redacted_7517 : PMIOPort  Port=22  Side=Left
  Redacted_9903 : PMIOPort  Port=23  Side=Left
  Redacted_4196 : PMIOPort  Port=24  Side=Left
  Redacted_7593 : PMIOPort  Port=25  Side=Left
  Redacted_5814 : PMIOPort  Port=26  Side=Left
  connections:
  Redacted_5814/RConn1 -- Redacted_6273/RConn2 -- Redacted_6455/RConn1
  Redacted_4691/LConn1 -- Redacted_8218/RConn1 -- Redacted_4691/LConn2
  Redacted_1895/RConn1 -- Redacted_3953/LConn1 -- Redacted_1905/LConn2
  Redacted_7361/RConn1 -- Redacted_105/RConn1 -- Redacted_4575/RConn2
  Redacted_5309/LConn2 -- Redacted_8680/LConn2 -- Redacted_2605/LConn2 -- Redacted_4547/LConn2 -- Redacted_7713/LConn2 -- Redacted_8952/LConn2 -- Redacted_1164/LConn2 -- Redacted_4638/LConn2 -- Redacted_5933/RConn1 -- Redacted_3416/LConn2
  Redacted_6511/LConn1 -- Redacted_1897/RConn1 -- Redacted_1488/LConn2
  Redacted_758/RConn2 -- Redacted_444/RConn1 -- Redacted_2216/RConn1
  Redacted_8218/LConn1 -- Redacted_5095/RConn1 -- Redacted_6212/LConn2
  Redacted_3408/RConn1 -- Redacted_672/LConn2 -- Redacted_672/LConn1
  Redacted_3208/RConn1 -- Redacted_5210/LConn2 -- Redacted_5210/LConn1
  Redacted_758/LConn1 -- Redacted_5529/RConn1 -- Redacted_2216/LConn2
  Redacted_2983/RConn1 -- Redacted_9833/LConn2 -- Redacted_9833/LConn1
  Redacted_4575/LConn1 -- Redacted_3718/RConn1 -- Redacted_7361/LConn2
  Redacted_3239/RConn1 -- Redacted_3619/LConn2 -- Redacted_3619/LConn1
  Redacted_6511/RConn2 -- Redacted_7138/RConn1 -- Redacted_1488/RConn1
  Redacted_758/RConn1 -- Redacted_28/LConn2 -- Redacted_28/LConn1
  Redacted_6511/RConn1 -- Redacted_8996/LConn2 -- Redacted_8996/LConn1
  Redacted_2151/RConn1 -- Redacted_302/LConn2 -- Redacted_302/LConn1
  Redacted_3953/RConn1 -- Redacted_8795/LConn2 -- Redacted_8795/LConn1
  Redacted_7816/RConn1 -- Redacted_3197/LConn2 -- Redacted_3197/LConn1
  Redacted_181/RConn1 -- Redacted_4191/LConn2 -- Redacted_4191/LConn1
  Redacted_8218/RConn2 -- Redacted_5373/RConn1 -- Redacted_6212/RConn1
  Redacted_4575/RConn1 -- Redacted_3093/LConn2 -- Redacted_3093/LConn1
  Redacted_9052/RConn1 -- Redacted_4798/RConn1 -- Redacted_3239/RConn2
  Redacted_4399/RConn1 -- Redacted_3239/LConn1 -- Redacted_4798/LConn2
  Redacted_1135/LConn1 -- Redacted_1135/LConn2 -- Redacted_6273/RConn1
  Redacted_8300/RConn1 -- Redacted_6455/LConn2 -- Redacted_6273/LConn1
  Redacted_50/RConn1 -- Redacted_7715/LConn2 -- Redacted_2151/LConn1
  Redacted_1513/RConn1 -- Redacted_8044/LConn2 -- Redacted_3408/LConn1
  Redacted_4142/RConn1 -- Redacted_181/LConn1 -- Redacted_9378/LConn2
  Redacted_9072/RConn1 -- Redacted_7816/LConn1 -- Redacted_9879/LConn2
  Redacted_8330/RConn1 -- Redacted_2983/LConn1 -- Redacted_662/LConn2
  Redacted_7870/RConn1 -- Redacted_3208/LConn1 -- Redacted_4152/LConn2
  Redacted_7593/RConn1 -- Redacted_7715/RConn1 -- Redacted_2151/RConn2
  Redacted_7634/RConn1 -- Redacted_3208/RConn2 -- Redacted_4152/RConn1
  Redacted_7555/RConn1 -- Redacted_3953/RConn2 -- Redacted_1905/RConn1
  Redacted_6684/RConn1 -- Redacted_2983/RConn2 -- Redacted_662/RConn1
  Redacted_7517/RConn1 -- Redacted_7816/RConn2 -- Redacted_9879/RConn1
  Redacted_9903/RConn1 -- Redacted_181/RConn2 -- Redacted_9378/RConn1
  Redacted_4196/RConn1 -- Redacted_3408/RConn2 -- Redacted_8044/RConn1
  Redacted_3197/RConn1 -- Redacted_4547/LConn1
  Redacted_672/RConn1 -- Redacted_8952/LConn1
  Redacted_3093/RConn1 -- Redacted_5733/LConn1
  Redacted_2216/LConn1 -- Redacted_3397/RConn1
  Redacted_4191/RConn1 -- Redacted_7713/LConn1
  Redacted_1905/LConn1 -- Redacted_8680/RConn1
  Redacted_4532/RConn1 -- Redacted_3397/LConn2
  Redacted_3619/RConn1 -- Redacted_3416/LConn1
  Redacted_4798/LConn1 -- Redacted_3416/RConn1
  Redacted_5210/RConn1 -- Redacted_5309/LConn1
  Redacted_4691/RConn1 -- Redacted_6084/LConn1
  Redacted_662/LConn1 -- Redacted_2605/RConn1
  Redacted_9833/RConn1 -- Redacted_2605/LConn1
  Redacted_28/RConn1 -- Redacted_3397/LConn1
  Redacted_9983/RConn1 -- Redacted_6084/LConn2
  Redacted_5309/RConn1 -- Redacted_4152/LConn1
  Redacted_1164/RConn1 -- Redacted_7715/LConn1
  Redacted_1488/LConn1 -- Redacted_998/RConn1
  Redacted_302/RConn1 -- Redacted_1164/LConn1
  Redacted_8795/RConn1 -- Redacted_8680/LConn1
  Redacted_8996/RConn1 -- Redacted_998/LConn1
  Redacted_8044/LConn1 -- Redacted_8952/RConn1
  Redacted_998/LConn2 -- Redacted_2039/RConn1
  Redacted_7361/LConn1 -- Redacted_5733/RConn1
  Redacted_6084/RConn1 -- Redacted_6212/LConn1
  Redacted_7713/RConn1 -- Redacted_9378/LConn1
  Redacted_5733/LConn2 -- Redacted_1339/RConn1
  Redacted_9879/LConn1 -- Redacted_4547/RConn1
  Redacted_1135/RConn1 -- Redacted_4638/LConn1
  Redacted_4638/RConn1 -- Redacted_6455/LConn1

== system Electrical_System_2018b_obfs/Redacted_1750/Redacted_3116/Redacted_9404 ==
  Redacted_3537 : fl_ps_legacy_lib/Legacy Physical Signals/Functions/PS Product
      settings: SourceProductName=Simscape  SourceProductBaseCode=SS
  Redacted_8032 : fl_lib/Electrical/Electrical Elements/Variable Resistor  Rmin=sbjxdqwimd Ohm  i_specify=off  i_priority=None  i=kzoqwsyddo A  i_nominal_specify=off  i_nominal_unit=A  i_nominal_value=ognfttygpz  v_specify=off  v_priority=None  v=rgbeapnhqb V  v_nominal_specify=off  v_nominal_unit=V  v_nominal_value=dvocgkuiiq
  Redacted_8913 : fl_lib/Physical Signals/Sources/PS Constant  constant=dewamaawgx
  Redacted_9130 : fl_ps_legacy_lib/Legacy Physical Signals/Functions/PS Divide
      settings: SourceProductName=Simscape  SourceProductBaseCode=SS  InternalSimscapePortConfiguration="{\"Bottom\":[],\"Left\":[{\"id\":\"I1\",\"label\":\"\",\"type\":\"input\"},{\"id\":\"I2\",\"label\":\"\",\"type\":\"input\"}],\"Right\":[{\"id\":\"O\",\"label\":\"\",\"type\":\"output\"}],\"Top\":[]}"
  Redacted_9338 : fl_lib/Electrical/Electrical Sensors/Voltage Sensor
  Redacted_6078 : PMIOPort  Side=Left
  Redacted_7382 : PMIOPort  Port=2  Side=Left
  connections:
  Redacted_8032/RConn1 -- Redacted_7382/RConn1 -- Redacted_9338/RConn2
  Redacted_9338/RConn1 -- Redacted_3537/LConn2 -- Redacted_3537/LConn1
  Redacted_8032/LConn2 -- Redacted_6078/RConn1 -- Redacted_9338/LConn1
  Redacted_9130/LConn2 -- Redacted_8913/RConn1
  Redacted_3537/RConn1 -- Redacted_9130/LConn1
  Redacted_9130/RConn1 -- Redacted_8032/LConn1
